simulink model "lab_1_4"  (R2023b)
settings: Solver=FixedStepAuto  StartTime=0.0  StopTime=10.0  FixedStep=0.001  RelTol=1e-3
settings Model: Creator=nsukh  LastModifiedBy=nsukh

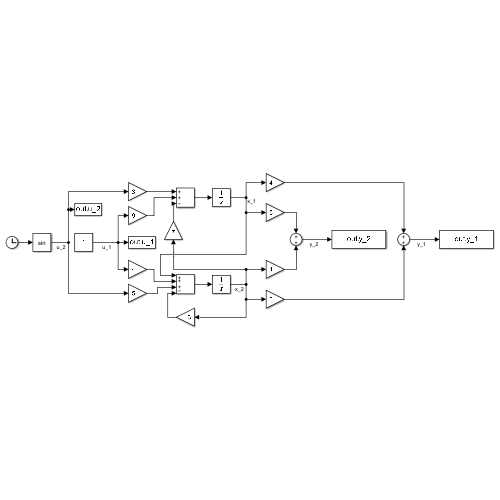
[thumbnail: Simulink's stored preview of the top-level diagram]
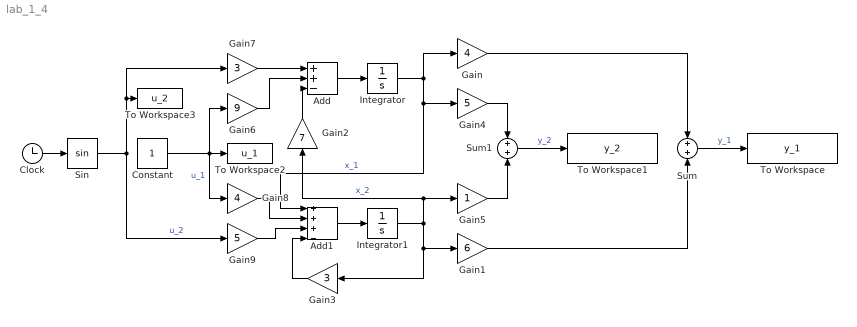
== system lab_1_4 ==
  Add : Sum  Inputs=++-
  Add1 : Sum  Inputs=+++-
  Clock : Clock
  Constant : Constant  SampleTime=-1
  Gain : Gain  Gain=4
  Gain1 : Gain  Gain=6
  Gain2 : Gain  Gain=7
  Gain3 : Gain  Gain=3
  Gain4 : Gain  Gain=5
  Gain5 : Gain
  Gain6 : Gain  Gain=9
  Gain7 : Gain  Gain=3
  Gain8 : Gain  Gain=4
  Gain9 : Gain  Gain=5
  Integrator : Integrator
  Integrator1 : Integrator
  Sin : Trigonometry
  Sum : Sum  Inputs=+|+
  Sum1 : Sum  Inputs=+|+
  To Workspace : ToWorkspace  VariableName=y_1  SaveFormat=Timeseries  SampleTime=-1
  To Workspace1 : ToWorkspace  VariableName=y_2  SaveFormat=Timeseries  SampleTime=-1
  To Workspace2 : ToWorkspace  VariableName=u_1  SaveFormat=Timeseries  SampleTime=-1
  To Workspace3 : ToWorkspace  VariableName=u_2  SaveFormat=Timeseries  SampleTime=-1
  wires:
  Clock/1 -> Sin/1
  Gain/1 -> Sum/1
  Gain1/1 -> Sum/2
  Sum/1 -> To Workspace/1  "y_1"
  Gain5/1 -> Sum1/2
  Gain4/1 -> Sum1/1
  Sum1/1 -> To Workspace1/1  "y_2"
  Integrator/1 -> Add1/1, Gain4/1, Gain/1  "x_1"
  Integrator1/1 -> Gain3/1, Gain1/1, Gain2/1, Gain5/1  "x_2"
  Add/1 -> Integrator/1
  Add1/1 -> Integrator1/1
  Gain2/1 -> Add/3
  Gain3/1 -> Add1/4
  Constant/1 -> To Workspace2/1, Gain6/1, Gain8/1  "u_1"
  Sin/1 -> Gain9/1, To Workspace3/1, Gain7/1  "u_2"
  Gain8/1 -> Add1/2
  Gain9/1 -> Add1/3
  Gain7/1 -> Add/1
  Gain6/1 -> Add/2
